simulink model "sim_rampa"  (R2018b)
settings: Solver=VariableStepAuto  StartTime=0.0  StopTime=2.34  RelTol=1e-3
undefined symbols (not defined in the file or in its folder): a, alpha, b, beta, den, dt, kd, kp, num
libraries: cstblocks x1, simulink_extras x1
settings Model: Creator=sergipetec  LastModifiedBy=sergipetec

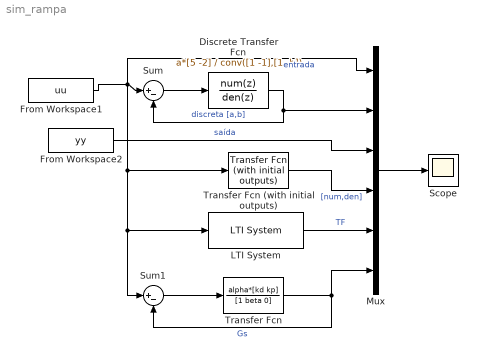
== system sim_rampa ==
  Discrete Transfer Fcn : DiscreteTransferFcn  Numerator=a*[5 -2]  Denominator=conv([1 -1],[1 -b])  SampleTime=dt
  From Workspace1 : FromWorkspace  VariableName=uu  SampleTime=dt
  From Workspace2 : FromWorkspace  VariableName=yy  SampleTime=dt
  LTI System : cstblocks/LTI System  sys=TF  IC=[]
  Mux : Mux  Inputs=6
  Scope : Scope
  Sum : Sum  Inputs=|+-
  Sum1 : Sum  Inputs=|+-
  Transfer Fcn : TransferFcn  Numerator=alpha*[kd kp]  Denominator=[1 beta 0]
  Transfer Fcn (with initial outputs) : simulink_extras/Additional Linear/Transfer Fcn (with initial outputs)  N=num  D=den  Y0=0  U0=0
  wires:
  From Workspace1/1 -> Mux/1, Sum1/1, LTI System/1, Transfer Fcn (with initial outputs)/1, Sum/1  "entrada"
  Discrete Transfer Fcn/1 -> Mux/2, Sum/2  "discreta [a,b]"
  Mux/1 -> Scope/1
  Sum/1 -> Discrete Transfer Fcn/1
  Sum1/1 -> Transfer Fcn/1
  Transfer Fcn/1 -> Mux/6, Sum1/2  "Gs"
  From Workspace2/1 -> Mux/3  "saída"
  LTI System/1 -> Mux/5  "TF"
  Transfer Fcn (with initial outputs)/1 -> Mux/4  "[num,den]"
